simulink model "WheelDriveModel"  (R2022a)
settings: Solver=VariableStepAuto  StartTime=0.0  StopTime=600  MaxStep=0.1  RelTol=1e-3
values from neighbouring files (symbols this model uses):
  gear_ratio = input_torque/(17.5*10^-3)    (= 134.4)    [SYDE351Project.m]
  input_torque = 9.8*mass_loaded*wheel_radius*0.6    (= 2.352)    [SYDE351Project.m]
  wheel_radius = 0.01    [SYDE351Project.m]
  wheel_separation = 0.5    [SYDE351Project.m]
settings Model: Creator=Bronz  LastModifiedBy=Bronz

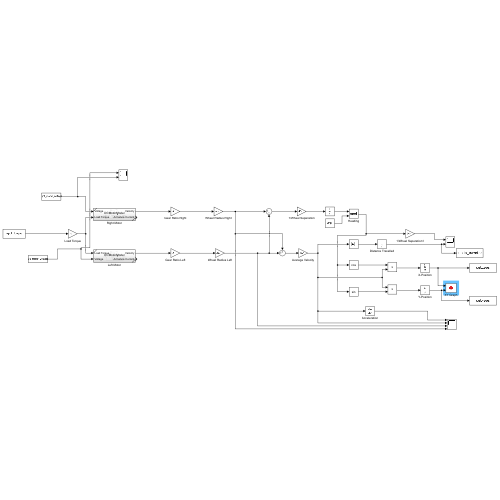
[thumbnail: Simulink's stored preview of the top-level diagram]
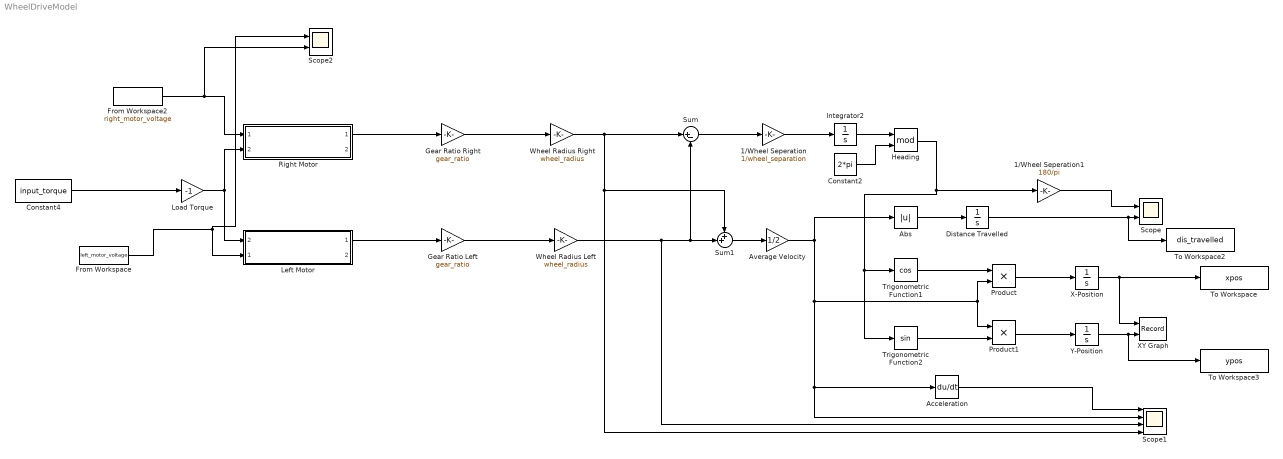
== system WheelDriveModel ==
  1/Wheel Seperation : Gain  Gain=1/wheel_separation
  1/Wheel Seperation1 : Gain  Gain=180/pi
  Abs : Abs  SaturateOnIntegerOverflow=off
  Acceleration : Derivative
  Average Velocity : Gain  Gain=1/2
  Constant2 : Constant  Value=2*pi
  Constant4 : Constant  Value=input_torque
  Distance Travelled : Integrator
  From Workspace : FromWorkspace  VariableName=left_motor_voltage
  From Workspace2 : FromWorkspace  VariableName=right_motor_voltage
  Gear Ratio Left : Gain  Gain=gear_ratio
  Gear Ratio Right : Gain  Gain=gear_ratio
  Heading : Math  Operator=mod
  Integrator2 : Integrator
  Left Motor : Subsystem  ReferencedSubsystem=DCMotorModel
      settings: PortSchema="{\"entries\":[{\"content\":{\"sides\":[{\"content\":{\"connectorIds\":[\"In2\",\"In1\"]},\"type\":\"ConnectorPlacement.EquallySpacedRectSide\",\"uuid\":\"328afdc4-2910-4488-afe5-6c44e5b70001\"},{\"content\":{\"connectorIds\":[\"Out1\",\"Out2\"],\"side\":\"RIGHT\"},\"type\":\"ConnectorPlacement.EquallySpacedRectSide\",\"uuid\":\"1cce0780-4cf2-4101-aaba-6ee003d6891f\"},{\"content\":{\"connectorIds\":[],\"side\":\"TOP\"},\"type\":\"ConnectorPlacement.EquallySpacedRectSide\",\"uuid\":\"9a07b49b-17b9-4d38-8d6b-3ebbc6b935cd\"}]},\"type\":\"ConnectorPlacement.EquallySpacedConnector\",\"uuid\":\"66c53b9e-1903-4c6b-b136-59f3c493ba0a\"}],\"packageUris\":[\"http://schema.mathworks.com/mf0/Connector/R2020b\"],\"version\":\"1.0\"}"
  Load Torque : Gain  Gain=-1
  Product : Product
  Product1 : Product
  Right Motor : Subsystem  ReferencedSubsystem=DCMotorModel
  Scope : Scope  NumInputPorts=2
  Scope1 : Scope  NumInputPorts=4
  Scope2 : Scope  NumInputPorts=2
  Sum : Sum  Inputs=|+-
  Sum1 : Sum  Inputs=++|
  To Workspace : ToWorkspace  VariableName=xpos  SaveFormat=Timeseries  SampleTime=-1
  To Workspace2 : ToWorkspace  VariableName=dis_travelled  SaveFormat=Timeseries  SampleTime=-1
  To Workspace3 : ToWorkspace  VariableName=ypos  SaveFormat=Timeseries  SampleTime=-1
  Trigonometric Function1 : Trigonometry  Operator=cos
  Trigonometric Function2 : Trigonometry
  Wheel Radius Left : Gain  Gain=wheel_radius
  Wheel Radius Right : Gain  Gain=wheel_radius
  X-Position : Integrator
  XY Graph : Record  FileSettingsInternal="{\"entries\":[{\"content\":{\"excelSettings\":{\"content\":{},\"type\":\"Streamout.ExcelSettings\"}},\"type\":\"Streamout.FileSettingStorage\",\"uuid\":\"33098972-c605-4ea9-8aa1-138a1e32de8d\"}],\"packageUris\":[\"http://schema.mathworks.com/mf0/streamout_blocks/R2020a\"],\"version\":\"1.0\"}"  Layout=[1 1]  SignalsInternal="{\"entries\":[{\"content\":{\"signals\":[{\"content\":{\"blockPath\":[\"WheelDriveModel/XY Graph\"],\"channel\":[],\"dimensions\":[1],\"domain\":\"WheelDriveModel/XY Graph\",\"lineColor\":\"#a2142f\",\"plots\":[1],\"port\":1,\"sid\":[\"\"],\"signalID\":4617,\"signalName\":\"X-Position\"},\"type\":\"RecordBlkView.Signal\",\"uuid\":\"5d654ee1-9bee-40d0-bc18-67a2da75a092\"},{\"content\":{\"blockPath\":[\"WheelDriveModel/XY Graph\"],\"channel\":[],\"dimensions\":[1],\"domain\":\"WheelDriveModel/XY Graph\",\"lineColor\":\"#139fff\",\"plots\":[1],\"port\":2,\"sid\":[\"\"],\"signalID\":4621,\"signalName\":\"Y-Position\"},\"type\":\"RecordBlkView.Signal\",\"uuid\":\"382f9a4c-99f0-47dd-ba25-88ed781a0ba1\"}]},\"type\":\"RecordBlkView.InputSignals\",\"uuid\":\"7ba725ef-0009-4a93-83d7-4d04a935a71c\"}],\"packageUris\":[\"http://schema.mathworks.com/mf0/streamout_blocks/R2020a\"],\"version\":\"1.0\"}"  VisualizationBindings="{\"xyplotplugin\":{\"info\":[{\"series\":[{\"bindingParametersList\":[{\"parameter\":\"X-Axis\",\"signalID\":4617,\"signalName\":\"X-Position\"},{\"parameter\":\"Y-Axis\",\"signalID\":4621,\"signalName\":\"Y-Position\"}],\"seriesID\":48845}],\"subplotID\":1}]}}"  CompatibilityTag=XY
  Y-Position : Integrator
  wires:
  Sum1/1 -> Average Velocity/1
  Average Velocity/1 -> Abs/1, Scope1/2, Acceleration/1, Product1/1, Product/2
  Distance Travelled/1 -> To Workspace2/1, Scope/2
  Product/1 -> X-Position/1
  X-Position/1 -> To Workspace/1, XY Graph/1
  Y-Position/1 -> To Workspace3/1, XY Graph/2
  Product1/1 -> Y-Position/1
  Trigonometric Function1/1 -> Product/1
  Trigonometric Function2/1 -> Product1/2
  Abs/1 -> Distance Travelled/1
  Acceleration/1 -> Scope1/1
  1/Wheel Seperation/1 -> Integrator2/1
  Sum/1 -> 1/Wheel Seperation/1
  Heading/1 -> Trigonometric Function2/1, Trigonometric Function1/1, 1/Wheel Seperation1/1
  Integrator2/1 -> Heading/1
  Constant2/1 -> Heading/2
  Load Torque/1 -> Left Motor/2, Right Motor/2
  Wheel Radius Right/1 -> Scope1/4, Sum1/1, Sum/1
  Wheel Radius Left/1 -> Scope1/3, Sum/2, Sum1/2
  Right Motor/1 -> Gear Ratio Right/1
  Gear Ratio Right/1 -> Wheel Radius Right/1
  Left Motor/1 -> Gear Ratio Left/1
  Gear Ratio Left/1 -> Wheel Radius Left/1
  From Workspace2/1 -> Scope2/2, Right Motor/1
  From Workspace/1 -> Scope2/1, Left Motor/1
  1/Wheel Seperation1/1 -> Scope/1
  Constant4/1 -> Load Torque/1
